simulink model "BANSHEE"  (Simulink 8.1)
settings: Solver=ode1  StartTime=0.0  StopTime=inf  FixedStep=Ts  MaxStep=1e-3  RelTol=1e-3
PostLoadFcn:
  | BANSHEE_init;
InitFcn:
  | BANSHEE_init;
undefined symbols (not defined in the file): Acid, Banshee_HWCtrl_IOs, Banshee_SEL751_Woodward_lib, DMS_slave_lib, DMSCommands, F1, F2, F3, fdesignblkfcn, Feeder1_lib, Feeder2_lib, Feeder3_lib, gcbh, generic_ethernet_cb, Lead, Left, relay_housing_lib, SM_UtilityService, SS_F1_RELAY_HOUSING, SS_F2_RELAY_HOUSING, SS_F3_RELAY_HOUSING, SS_Feeder1, SS_Feeder2, SS_Feeder3, SUBSTATION, TestSeq_slave_lib, TestSequenceCommands, Ts, type, utility_service_lib, V
libraries: powerlib x106, cables_lib x61, breaker_lib x53, rtio_generic_modbus x50, relay_modbus_lib x45, rtio_opalrt_op5142ex1 x37, transformer_lib x29, rteventslib x28, simulink x24, Load_lib x24, rtlab x20, ssn_lib x19
(part 8 of 9)

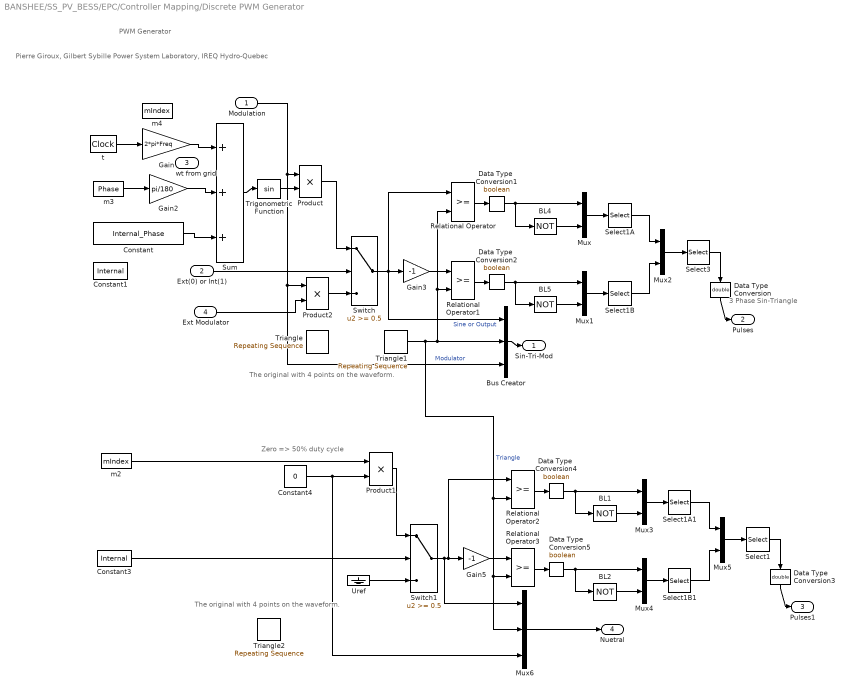
== system BANSHEE/SS_PV_BESS/EPC/Controller Mapping/Discrete PWM Generator ==
  note: Pierre Giroux, Gilbert Sybille
      | Power System Laboratory, IREQ
      | Hydro-Quebec
  note: PWM Generator
  note: 3 Phase
      | Sin-Triangle
  note: Zero => 50% duty cycle
  note: The original with 4
      | points on the waveform.
  note: The original with 4
      | points on the waveform.
  Modulation : Inport
  Ext(0) or Int(1) : Inport  Port=2
  wt from grid : Inport  Port=3
  Ext Modulator : Inport  Port=4
  BL{1..2,4..5} (4 alike) : Logic  Operator=NOT  Inputs=1  SampleTime=Ts
  Bus Creator : BusCreator  Inputs=3
  Constant : Constant  Value=Internal_Phase  SampleTime=Ts
  Constant1 : Constant  Value=Internal  SampleTime=Ts
  Constant3 : Constant  Value=Internal  SampleTime=Ts
  Constant4 : Constant  Value=0
  Data Type  Conversion : DataTypeConversion  OutDataTypeStr=double  SampleTime=Ts  SaturateOnIntegerOverflow=on  RndMeth=Zero
  Data Type  Conversion{1..2,4..5} (4 alike) : DataTypeConversion  OutDataTypeStr=boolean  SampleTime=Ts  SaturateOnIntegerOverflow=on  RndMeth=Zero
  Data Type  Conversion3 : DataTypeConversion  OutDataTypeStr=double  SampleTime=Ts  SaturateOnIntegerOverflow=on  RndMeth=Zero
  Gain : Gain  Gain=2*pi*Freq  SaturateOnIntegerOverflow=on  OutDataTypeStr=Inherit: Same as input  ParamDataTypeStr=Inherit: Same as input
  Gain2 : Gain  Gain=pi/180  SaturateOnIntegerOverflow=on  OutDataTypeStr=Inherit: Same as input  ParamDataTypeStr=Inherit: Same as input
  Gain3 : Gain  Gain=-1  SampleTime=Ts  SaturateOnIntegerOverflow=on  OutDataTypeStr=Inherit: Same as input  ParamDataTypeStr=Inherit: Same as input
  Gain5 : Gain  Gain=-1  SampleTime=Ts  SaturateOnIntegerOverflow=on  OutDataTypeStr=Inherit: Same as input  ParamDataTypeStr=Inherit: Same as input
  Mux{,1..5} (6 alike) : Mux  Inputs=2
  Mux6 : Mux  Inputs=3
  Product : Product  SampleTime=Ts  SaturateOnIntegerOverflow=on  InputSameDT=on  OutDataTypeStr=Inherit: Same as first input
  Product1 : Product  SampleTime=Ts  SaturateOnIntegerOverflow=on  InputSameDT=on  OutDataTypeStr=Inherit: Same as first input
  Product2 : Product  SampleTime=Ts  SaturateOnIntegerOverflow=on  InputSameDT=on  OutDataTypeStr=Inherit: Same as first input
  Relational Operator{,1..3} (4 alike) : RelationalOperator  SampleTime=Ts  InputSameDT=on
  Select1 : Selector  InputPortWidth=Select3_PortWidth  IndexOptions=Index vector (dialog)  Indices=Select3_Elements  OutputSizes=1
  Select1A : Selector  InputPortWidth=Select1_PortWidth  IndexOptions=Index vector (dialog)  Indices=Select1_Elements  OutputSizes=1
  Select1A1 : Selector  InputPortWidth=Select1_PortWidth  IndexOptions=Index vector (dialog)  Indices=Select1_Elements  OutputSizes=1
  Select1B : Selector  InputPortWidth=Select1_PortWidth  IndexOptions=Index vector (dialog)  Indices=Select1_Elements  OutputSizes=1
  Select1B1 : Selector  InputPortWidth=Select1_PortWidth  IndexOptions=Index vector (dialog)  Indices=Select1_Elements  OutputSizes=1
  Select3 : Selector  InputPortWidth=Select3_PortWidth  IndexOptions=Index vector (dialog)  Indices=Select3_Elements  OutputSizes=1
  Sum : Sum  Inputs=+++  SampleTime=Ts  SaturateOnIntegerOverflow=on  InputSameDT=on  OutDataTypeStr=Inherit: Same as first input
  Switch : Switch  Threshold=0.5  SampleTime=Ts  SaturateOnIntegerOverflow=on  InputSameDT=on
  Switch1 : Switch  Threshold=0.5  SampleTime=Ts  SaturateOnIntegerOverflow=on  InputSameDT=on
  Triangle : simulink/Sources/Repeating Sequence  rep_seq_t=[0 1/Fc/4 3/Fc/4 1/Fc]  rep_seq_y=[0 -1 1 0]
  Triangle1 : simulink/Sources/Repeating Sequence  rep_seq_t=[0 1/Fc/2 1/Fc]  rep_seq_y=[-1 1 -1]
  Triangle2 : simulink/Sources/Repeating Sequence  rep_seq_t=[0 1/Fc/4 3/Fc/4 1/Fc]  rep_seq_y=[0 -1 1 0]
  Trigonometric Function : Trigonometry  SampleTime=Ts
  Uref : Ground
  m2 : Constant  Value=mIndex  SampleTime=Ts
  m3 : Constant  Value=Phase  SampleTime=Ts
  m4 : Constant  Value=mIndex  SampleTime=Ts
  t : DigitalClock  SampleTime=Ts
  Sin-Tri-Mod : Outport  SampleTime=Ts
  Pulses : Outport  Port=2  SampleTime=Ts
  Pulses1 : Outport  Port=3  SampleTime=Ts
  Nuetral : Outport  Port=4  SampleTime=Ts
  wires:
  Switch/1 -> Relational Operator/1, Gain3/1, Bus Creator/1  "Sine or Output"
  Mux2/1 -> Select3/1
  Select1B/1 -> Mux2/2
  Select1A/1 -> Mux2/1
  Mux1/1 -> Select1B/1
  Mux/1 -> Select1A/1
  BL5/1 -> Mux1/2
  BL4/1 -> Mux/2
  Gain3/1 -> Relational Operator1/1
  Product/1 -> Switch/1
  Trigonometric Function/1 -> Product/2
  Sum/1 -> Trigonometric Function/1
  m3/1 -> Gain2/1
  t/1 -> Gain/1
  Select3/1 -> Data Type  Conversion/1
  Data Type  Conversion/1 -> Pulses/1
  Relational Operator/1 -> Data Type  Conversion1/1
  Data Type  Conversion1/1 -> BL4/1, Mux/1
  Relational Operator1/1 -> Data Type  Conversion2/1
  Data Type  Conversion2/1 -> BL5/1, Mux1/1
  Bus Creator/1 -> Sin-Tri-Mod/1
  Triangle1/1 -> Bus Creator/2, Relational Operator1/2, Relational Operator/2, Relational Operator3/2, Mux6/2, Relational Operator2/2  "Triangle"
  Switch1/1 -> Relational Operator2/1, Gain5/1, Mux6/1
  Mux5/1 -> Select1/1
  Select1B1/1 -> Mux5/2
  Select1A1/1 -> Mux5/1
  Mux4/1 -> Select1B1/1
  Mux3/1 -> Select1A1/1
  BL2/1 -> Mux4/2
  BL1/1 -> Mux3/2
  Gain5/1 -> Relational Operator3/1
  Product1/1 -> Switch1/1
  m2/1 -> Product1/1
  Select1/1 -> Data Type  Conversion3/1
  Data Type  Conversion3/1 -> Pulses1/1
  Relational Operator2/1 -> Data Type  Conversion4/1
  Data Type  Conversion4/1 -> BL1/1, Mux3/1
  Relational Operator3/1 -> Data Type  Conversion5/1
  Data Type  Conversion5/1 -> BL2/1, Mux4/1
  Constant4/1 -> Product1/2, Mux6/3
  Mux6/1 -> Nuetral/1
  Product2/1 -> Switch/3
  Constant3/1 -> Switch1/2
  Uref/1 -> Switch1/3
  Ext(0) or Int(1)/1 -> Switch/2
  Modulation/1 -> Bus Creator/3, Product2/1, Product/1  "Modulator"
  Ext Modulator/1 -> Product2/2
  Constant/1 -> Sum/3
  Gain2/1 -> Sum/2
  Gain/1 -> Sum/1

== system BANSHEE/SS_PV_BESS/EPC/Controller Mapping/EPC Inverter Controller Outputs ==
  note: These PWM IN Signals will be used.
      | PWM 1 and 2 are Bot and Top
      | PWM 3 and 4 are Bot and Top
      | PWM 5 and 6 are Bot and Top
  note: When using TSD set the DOUT type config to 0
      | When using PWM set the DOUT type config to 1
  note: It was at 1 for PWM, but it seems that
      | it is better to use the event detector conversion
      | block with TSD instead.
  note: % Copyright (c) 2016 Massachusetts Institute of Technology
      | % Permission is hereby granted, free of charge, to any person obtaining a copy of this
      | % software and associated documentation files (the "Software"), to deal in the Software
      | % without restriction, including without limitation the rights to use, copy, modify,
      | % merge, publish, distribute, sublicense, and/or sell copies of the Software, and to
      | % permit persons to whom the Software is furnished to do so, subject to the following
      | % conditions:
      | %
      | %
      | % The above copyright notice and this permission notice shall be included in
      | % all copies or substantial portions of the Software.
      | %
      | % THE SOFTWARE IS PROVIDED "AS IS", WITHOUT WARRANTY OF ANY KIND, EXPRESS OR IMPLIED,
      | % INCLUDING BUT NOT LIMITED TO THE WARRANTIES OF MERCHANTABILITY, FITNESS FOR A
      | % PARTICULAR PURPOSE AND NONINFRINGEMENT. IN NO EVENT SHALL THE AUTHORS OR COPYRIGHT
      | % HOLDERS BE LIABLE FOR ANY CLAIM, DAMAGES OR OTHER LIABILITY, WHETHER IN AN ACTION
      | % OF CONTRACT, TORT OR OTHERWISE, ARISING FROM, OUT OF OR IN CONNECTION WITH THE
      | % SOFTWARE OR THE USE OR OTHER DEALINGS IN THE SOFTWARE.
      | %
      | %
      | %%
  Console Input : Inport
  Bus Creator1 : BusCreator  Inputs=3
  Bus Creator2 : BusCreator  Inputs=2
  Bus Selector1 : BusSelector  OutputSignals=00-03,04-07  OutputAsBus=on
  Bus Selector2 : BusSelector  OutputSignals=08-11,12-15  OutputAsBus=on
  Bus Selector6 : BusSelector  OutputSignals=16 DOUT GR3,16 TSDOUT GR3,16 PWMOUT GR3
  DIO - Gr4 : Subsystem
  DOUT type config : Subsystem
  GR1 B AIN (CH00-15) : Subsystem
  OpCtrl OP5142EX2 : rtio_opalrt_op5142ex1/OpCtrl OP5142EX1  CtrlName='OP5142EX2 Ctrl'  boardid=2  BitstreamFilename=OP5142_1-EX-0000-2_3_4_54-16AIO_48AO_16DIO_16selDIO_CD-FF-01.bin  numconfig=-1  mode=Slave  externalClock=off  decimRtsi=0  calibIO=off  SampleTime=0  loadinport=-1
  PWM IO - Gr4 : Subsystem
  TSDIO - Gr4 : Subsystem
  Error : Outport
  IDs : Outport  Port=2
  PWM : Outport  Port=3
  Digital Inputs : Outport  Port=4
  PWM_RTE : Outport  Port=5
  BESS_TSD_RTE : Outport  Port=6
  PV_TSD_RTE : Outport  Port=7
  wires:
  TSDIO - Gr4/3(PV_TSDin_RTE) -> PV_TSD_RTE/1
  OpCtrl OP5142EX2/1 -> Error/1
  OpCtrl OP5142EX2/2 -> IDs/1
  PWM IO - Gr4/1(PWMIn) -> Bus Creator1/3, PWM/1  "PWMIN"
  TSDIO - Gr4/1(TSDin) -> Bus Creator1/2  "TSDIN"
  DIO - Gr4/1(DIn) -> Bus Creator1/1  "DIN"
  Bus Creator1/1 -> Digital Inputs/1
  Console Input/1 -> Bus Selector6/1
  Bus Selector6/2 -> TSDIO - Gr4/1(TSDout)  "<16 TSDOUT GR3>"
  Bus Selector6/3 -> PWM IO - Gr4/1(PWMOut)  "<16 PWMOUT GR3>"
  Bus Selector6/1 -> Bus Selector1/1, Bus Selector2/1  "<16 DOUT GR3>"
  Bus Selector1/1 -> Bus Creator2/1  "DI_CH00-07"
  Bus Selector2/1 -> Bus Creator2/2  "DI_CH08-15"
  Bus Creator2/1 -> DIO - Gr4/1(Dout)
  PWM IO - Gr4/2(PWMIn_RTE) -> PWM_RTE/1
  TSDIO - Gr4/2(BESS_TSDin_RTE) -> BESS_TSD_RTE/1

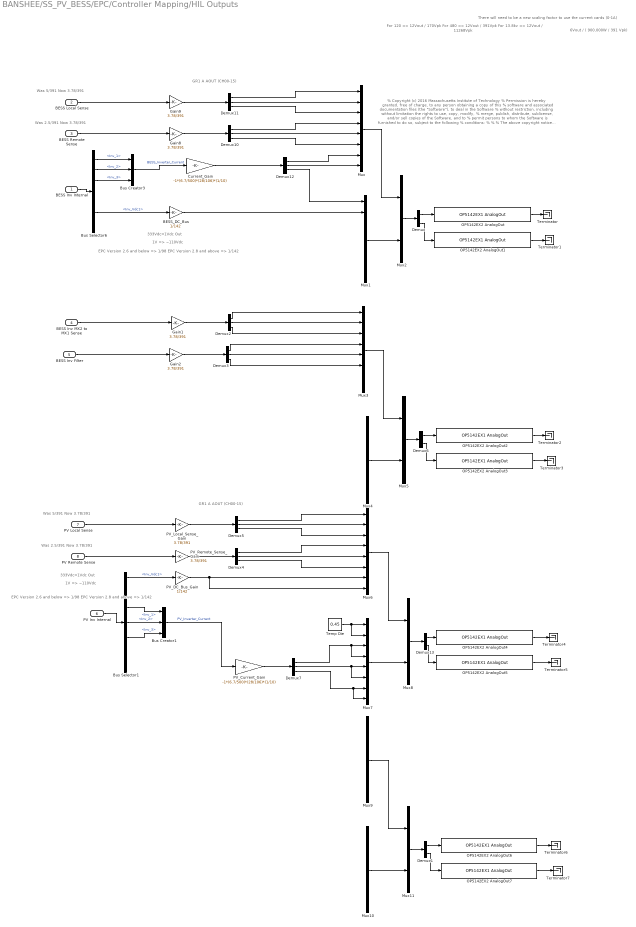
== system BANSHEE/SS_PV_BESS/EPC/Controller Mapping/HIL Outputs ==
  note: GR1 A AOUT (CH00-15)
  note: 333Vdc=1Vdc Out
  note: 1V => ~110Vdc
  note: Was 5/391
      | Now 3.78/391
  note: Was 2.5/391
      | Now 3.78/391
  note: EPC Version 2.6 and below => 1/98
      | EPC Version 2.8 and above => 1/142
  note: 6Vout / ( 900,000W / 391 Vpk)
  note: For 120 => 12Vout / 170Vpk
      | For 480 => 12Vout / 391Vpk
      | For 13.8kv => 12Vout / 11268Vpk
  note: GR1 A AOUT (CH00-15)
  note: There will need to be a
      | new scaling factor to use
      | the current cards (0-1A)
  note: 333Vdc=1Vdc Out
  note: 1V => ~110Vdc
  note: Was 5/391
      | Now 3.78/391
  note: Was 2.5/391
      | Now 3.78/391
  note: EPC Version 2.6 and below => 1/98
      | EPC Version 2.8 and above => 1/142
  note: % Copyright (c) 2016 Massachusetts Institute of Technology
      | % Permission is hereby granted, free of charge, to any person obtaining a copy of this
      | % software and associated documentation files (the "Software"), to deal in the Software
      | % without restriction, including without limitation the rights to use, copy, modify,
      | % merge, publish, distribute, sublicense, and/or sell copies of the Software, and to
      | % permit persons to whom the Software is furnished to do so, subject to the following
      | % conditions:
      | %
      | %
      | % The above copyright notice and this permission notice shall be included in
      | % all copies or substantial portions of the Software.
      | %
      | % THE SOFTWARE IS PROVIDED "AS IS", WITHOUT WARRANTY OF ANY KIND, EXPRESS OR IMPLIED,
      | % INCLUDING BUT NOT LIMITED TO THE WARRANTIES OF MERCHANTABILITY, FITNESS FOR A
      | % PARTICULAR PURPOSE AND NONINFRINGEMENT. IN NO EVENT SHALL THE AUTHORS OR COPYRIGHT
      | % HOLDERS BE LIABLE FOR ANY CLAIM, DAMAGES OR OTHER LIABILITY, WHETHER IN AN ACTION
      | % OF CONTRACT, TORT OR OTHERWISE, ARISING FROM, OUT OF OR IN CONNECTION WITH THE
      | % SOFTWARE OR THE USE OR OTHER DEALINGS IN THE SOFTWARE.
      | %
      | %
      | %%
  BESS Inv Internal : Inport
  BESS Local Sense : Inport  Port=2
  BESS Remote Sense : Inport  Port=3
  BESS Inv MX2 to MX1 Sense : Inport  Port=4
  BESS Inv Filter : Inport  Port=5
  PV Inv Internal : Inport  Port=6
  PV Local Sense : Inport  Port=7
  PV Remote Sense : Inport  Port=8
  BESS_DC_Bus : Gain  Gain=1/142
  Bus Creator1 : BusCreator  Inputs=3
  Bus Creator3 : BusCreator  Inputs=3
  Bus Selector1 : BusSelector  OutputSignals=Inv_Vdc1,Inv_Vdc2,Inv_1,Inv_2,Inv_3,Inv_Idc1,Inv_Idc2
  Bus Selector6 : BusSelector  OutputSignals=Inv_1,Inv_2,Inv_3,Inv_Idc1,Inv_Idc2,Inv_Vdc1,Inv_Vdc2
  Current_Gain : Gain  Gain=-1*(6.7/500)*(28/106)*(1/10)
  Demux{,1,6,13} (4 alike) : Demux  Outputs=2
  Demux{2..5,7,10..12} (8 alike) : Demux  Outputs=3
  Gain{1..2,8..9} (4 alike) : Gain  Gain=3.78/391
  Mux{,1,3..4,6..7,9..10} (8 alike) : Mux  Inputs=8
  Mux{2,5,8,11} (4 alike) : Mux  Inputs=2
  OP5142EX2 AnalogOut : rtio_opalrt_op5142ex1/OP5142EX1 AnalogOut  CtrlName='OP5142EX2 Ctrl'  portNb=1  FcnNos=Slot 1 Module A Subsection 1  size=16  maxcount=8  count=8  numchan=8  israngeinput=off  voltagerange=[-16 ... 16]  slot=0  side=0  mismatch=0  slotside=Slot_1_Module_A
      settings: AttributesFormatString=%<CtrlName>
  OP5142EX2 AnalogOut1 : rtio_opalrt_op5142ex1/OP5142EX1 AnalogOut  CtrlName='OP5142EX2 Ctrl'  portNb=2  FcnNos=Slot 1 Module A Subsection 2  size=16  maxcount=8  count=8  numchan=8  israngeinput=off  voltagerange=[-16 ... 16]  slot=0  side=0  mismatch=0  slotside=Slot_1_Module_A
      settings: AttributesFormatString=%<CtrlName>
  OP5142EX2 AnalogOut2 : rtio_opalrt_op5142ex1/OP5142EX1 AnalogOut  CtrlName='OP5142EX2 Ctrl'  portNb=3  FcnNos=Slot 2 Module A Subsection 1  size=16  maxcount=8  count=8  numchan=8  israngeinput=off  voltagerange=[-16 ... 16]  slot=1  side=0  mismatch=0  slotside=Slot_2_Module_A
      settings: AttributesFormatString=%<CtrlName>
  OP5142EX2 AnalogOut3 : rtio_opalrt_op5142ex1/OP5142EX1 AnalogOut  CtrlName='OP5142EX2 Ctrl'  portNb=4  FcnNos=Slot 2 Module A Subsection 2  size=16  maxcount=8  count=8  numchan=8  israngeinput=off  voltagerange=[-16 ... 16]  slot=1  side=0  mismatch=0  slotside=Slot_2_Module_A
      settings: AttributesFormatString=%<CtrlName>
  OP5142EX2 AnalogOut4 : rtio_opalrt_op5142ex1/OP5142EX1 AnalogOut  CtrlName='OP5142EX2 Ctrl'  portNb=5  FcnNos=Slot 2 Module B Subsection 1  size=16  maxcount=8  count=8  numchan=8  israngeinput=off  voltagerange=[-16 ... 16]  slot=1  side=1  mismatch=0  slotside=Slot_2_Module_B
      settings: AttributesFormatString=%<CtrlName>
  OP5142EX2 AnalogOut5 : rtio_opalrt_op5142ex1/OP5142EX1 AnalogOut  CtrlName='OP5142EX2 Ctrl'  portNb=6  FcnNos=Slot 2 Module B Subsection 2  size=16  maxcount=8  count=8  numchan=8  israngeinput=off  voltagerange=[-16 ... 16]  slot=1  side=1  mismatch=0  slotside=Slot_2_Module_B
      settings: AttributesFormatString=%<CtrlName>
  OP5142EX2 AnalogOut6 : rtio_opalrt_op5142ex1/OP5142EX1 AnalogOut  CtrlName='OP5142EX2 Ctrl'  portNb=7  FcnNos=Slot 3 Module A Subsection 1  size=16  maxcount=8  count=8  numchan=8  israngeinput=off  voltagerange=[-16 ... 16]  slot=2  side=0  mismatch=0  slotside=Slot_3_Module_A
      settings: AttributesFormatString=%<CtrlName>
  OP5142EX2 AnalogOut7 : rtio_opalrt_op5142ex1/OP5142EX1 AnalogOut  CtrlName='OP5142EX2 Ctrl'  portNb=8  FcnNos=Slot 3 Module A Subsection 2  size=16  maxcount=8  count=8  numchan=8  israngeinput=off  voltagerange=[-16 ... 16]  slot=2  side=0  mismatch=0  slotside=Slot_3_Module_A
      settings: AttributesFormatString=%<CtrlName>
  PV_Current_Gain : Gain  Gain=-1*(6.7/500)*(28/106)*(1/10)
  PV_DC_Bus_Gain : Gain  Gain=1/142
  PV_Local_Sense_Gain : Gain  Gain=3.78/391
  PV_Remote_Sense_Gain : Gain  Gain=3.78/391
  Temp Die : Constant  Value=0.45
  Terminator{,1..7} (8 alike) : Terminator
  wires:
  Temp Die/1 -> Mux7/1, Mux7/2
  Demux7/3 -> Mux7/7, Mux7/8
  Demux7/2 -> Mux7/5, Mux7/6
  Demux7/1 -> Mux7/3, Mux7/4
  Demux4/3 -> Mux6/6
  Demux4/1 -> Mux6/4
  Demux4/2 -> Mux6/5
  Demux5/3 -> Mux6/3
  Demux5/1 -> Mux6/1
  Demux5/2 -> Mux6/2
  PV_Current_Gain/1 -> Demux7/1
  PV_Remote_Sense_Gain/1 -> Demux4/1
  PV_Local_Sense_Gain/1 -> Demux5/1
  PV_DC_Bus_Gain/1 -> Mux6/8, Mux6/7
  PV Inv Internal/1 -> Bus Selector1/1
  PV Local Sense/1 -> PV_Local_Sense_Gain/1
  PV Remote Sense/1 -> PV_Remote_Sense_Gain/1
  Bus Creator1/1 -> PV_Current_Gain/1  "PV_Inverter_Current"
  Bus Selector1/3 -> Bus Creator1/1  "<Inv_1>"
  Bus Selector1/4 -> Bus Creator1/2  "<Inv_2>"
  Bus Selector1/5 -> Bus Creator1/3  "<Inv_3>"
  Bus Selector1/1 -> PV_DC_Bus_Gain/1  "<Inv_Vdc1>"
  Demux10/3 -> Mux/6
  Demux10/1 -> Mux/4
  Demux10/2 -> Mux/5
  Demux11/3 -> Mux/3
  Demux11/1 -> Mux/1
  Demux11/2 -> Mux/2
  Current_Gain/1 -> Demux12/1
  Mux2/1 -> Demux/1
  Mux1/1 -> Mux2/2
  Mux/1 -> Mux2/1
  Demux/2 -> OP5142EX2 AnalogOut1/1
  Demux/1 -> OP5142EX2 AnalogOut/1
  OP5142EX2 AnalogOut1/1 -> Terminator1/1
  OP5142EX2 AnalogOut/1 -> Terminator/1
  Mux5/1 -> Demux6/1
  Mux4/1 -> Mux5/2
  Mux3/1 -> Mux5/1
  Demux6/2 -> OP5142EX2 AnalogOut3/1
  Demux6/1 -> OP5142EX2 AnalogOut2/1
  OP5142EX2 AnalogOut3/1 -> Terminator3/1
  OP5142EX2 AnalogOut2/1 -> Terminator2/1
  Mux8/1 -> Demux13/1
  Mux7/1 -> Mux8/2
  Mux6/1 -> Mux8/1
  Gain8/1 -> Demux10/1
  Gain9/1 -> Demux11/1
  BESS_DC_Bus/1 -> Mux1/2
  BESS Inv Internal/1 -> Bus Selector6/1
  BESS Local Sense/1 -> Gain9/1
  BESS Remote Sense/1 -> Gain8/1
  Bus Creator3/1 -> Current_Gain/1  "BESS_Inverter_Current"
  Demux12/1 -> Mux/7
  Demux12/2 -> Mux/8
  Demux12/3 -> Mux1/1
  Bus Selector6/1 -> Bus Creator3/1  "<Inv_1>"
  Bus Selector6/2 -> Bus Creator3/2  "<Inv_2>"
  Bus Selector6/3 -> Bus Creator3/3  "<Inv_3>"
  Bus Selector6/6 -> BESS_DC_Bus/1  "<Inv_Vdc1>"
  Mux11/1 -> Demux1/1
  Mux10/1 -> Mux11/2
  Mux9/1 -> Mux11/1
  Demux13/1 -> OP5142EX2 AnalogOut4/1
  Demux13/2 -> OP5142EX2 AnalogOut5/1
  OP5142EX2 AnalogOut4/1 -> Terminator4/1
  OP5142EX2 AnalogOut5/1 -> Terminator5/1
  Demux1/1 -> OP5142EX2 AnalogOut6/1
  Demux1/2 -> OP5142EX2 AnalogOut7/1
  OP5142EX2 AnalogOut6/1 -> Terminator6/1
  OP5142EX2 AnalogOut7/1 -> Terminator7/1
  Gain1/1 -> Demux2/1
  BESS Inv MX2 to MX1 Sense/1 -> Gain1/1
  Demux2/1 -> Mux3/1
  Demux2/2 -> Mux3/2
  Demux2/3 -> Mux3/3
  Gain2/1 -> Demux3/1
  BESS Inv Filter/1 -> Gain2/1
  Demux3/1 -> Mux3/4
  Demux3/2 -> Mux3/5
  Demux3/3 -> Mux3/6

== system BANSHEE/SS_PV_BESS/EPC/Controller Mapping/Mux to Pulses1 ==
  Mux_6_Pulses : Inport
  Bus Creator24 : BusCreator  Inputs=6
  Bus Selector5 : BusSelector  OutputSignals=Pulse 1,Pulse 2,Pulse 3,Pulse 4,Pulse 5,Pulse 6
  Demux5 : Demux  Outputs=6
  Pulse1 : Outport
  Pulse2 : Outport  Port=2
  Pulse3 : Outport  Port=3
  Pulse4 : Outport  Port=4
  Pulse5 : Outport  Port=5
  Pulse6 : Outport  Port=6
  Bus : Outport  Port=7
  wires:
  Demux5/1 -> Bus Creator24/1  "Pulse 1"
  Demux5/2 -> Bus Creator24/2  "Pulse 2"
  Demux5/3 -> Bus Creator24/3  "Pulse 3"
  Demux5/4 -> Bus Creator24/4  "Pulse 4"
  Demux5/5 -> Bus Creator24/5  "Pulse 5"
  Demux5/6 -> Bus Creator24/6  "Pulse 6"
  Bus Creator24/1 -> Bus Selector5/1, Bus/1
  Mux_6_Pulses/1 -> Demux5/1
  Bus Selector5/1 -> Pulse1/1  "<Pulse 1>"
  Bus Selector5/2 -> Pulse2/1  "<Pulse 2>"
  Bus Selector5/3 -> Pulse3/1  "<Pulse 3>"
  Bus Selector5/4 -> Pulse4/1  "<Pulse 4>"
  Bus Selector5/5 -> Pulse5/1  "<Pulse 5>"
  Bus Selector5/6 -> Pulse6/1  "<Pulse 6>"

== system BANSHEE/SS_PV_BESS/EPC/Controller Mapping/Mux to Pulses2 ==
  Mux_6_Pulses : Inport
  Bus Creator24 : BusCreator  Inputs=6
  Bus Selector5 : BusSelector  OutputSignals=Pulse 1,Pulse 2,Pulse 3,Pulse 4,Pulse 5,Pulse 6
  Demux5 : Demux  Outputs=6
  Pulse1 : Outport
  Pulse2 : Outport  Port=2
  Pulse3 : Outport  Port=3
  Pulse4 : Outport  Port=4
  Pulse5 : Outport  Port=5
  Pulse6 : Outport  Port=6
  Bus : Outport  Port=7
  wires:
  Demux5/1 -> Bus Creator24/1  "Pulse 1"
  Demux5/2 -> Bus Creator24/2  "Pulse 2"
  Demux5/3 -> Bus Creator24/3  "Pulse 3"
  Demux5/4 -> Bus Creator24/4  "Pulse 4"
  Demux5/5 -> Bus Creator24/5  "Pulse 5"
  Demux5/6 -> Bus Creator24/6  "Pulse 6"
  Bus Creator24/1 -> Bus Selector5/1, Bus/1
  Mux_6_Pulses/1 -> Demux5/1
  Bus Selector5/1 -> Pulse1/1  "<Pulse 1>"
  Bus Selector5/2 -> Pulse2/1  "<Pulse 2>"
  Bus Selector5/3 -> Pulse3/1  "<Pulse 3>"
  Bus Selector5/4 -> Pulse4/1  "<Pulse 4>"
  Bus Selector5/5 -> Pulse5/1  "<Pulse 5>"
  Bus Selector5/6 -> Pulse6/1  "<Pulse 6>"

== system BANSHEE/SS_PV_BESS/EPC/Controller Mapping/Mux to Pulses3 ==
  Mux_6_Pulses : Inport
  Bus Creator24 : BusCreator  Inputs=6
  Bus Selector5 : BusSelector  OutputSignals=Pulse 1,Pulse 2,Pulse 3,Pulse 4,Pulse 5,Pulse 6
  Demux5 : Demux  Outputs=6
  Pulse1 : Outport
  Pulse2 : Outport  Port=2
  Pulse3 : Outport  Port=3
  Pulse4 : Outport  Port=4
  Pulse5 : Outport  Port=5
  Pulse6 : Outport  Port=6
  Bus : Outport  Port=7
  wires:
  Demux5/1 -> Bus Creator24/1  "Pulse 1"
  Demux5/2 -> Bus Creator24/2  "Pulse 2"
  Demux5/3 -> Bus Creator24/3  "Pulse 3"
  Demux5/4 -> Bus Creator24/4  "Pulse 4"
  Demux5/5 -> Bus Creator24/5  "Pulse 5"
  Demux5/6 -> Bus Creator24/6  "Pulse 6"
  Bus Creator24/1 -> Bus Selector5/1, Bus/1
  Mux_6_Pulses/1 -> Demux5/1
  Bus Selector5/1 -> Pulse1/1  "<Pulse 1>"
  Bus Selector5/2 -> Pulse2/1  "<Pulse 2>"
  Bus Selector5/3 -> Pulse3/1  "<Pulse 3>"
  Bus Selector5/4 -> Pulse4/1  "<Pulse 4>"
  Bus Selector5/5 -> Pulse5/1  "<Pulse 5>"
  Bus Selector5/6 -> Pulse6/1  "<Pulse 6>"

== system BANSHEE/SS_PV_BESS/EPC/Controller Mapping/Mux to Pulses4 ==
  Mux_6_Pulses : Inport
  Bus Creator24 : BusCreator  Inputs=6
  Bus Selector5 : BusSelector  OutputSignals=Pulse 1,Pulse 2,Pulse 3,Pulse 4,Pulse 5,Pulse 6
  Demux5 : Demux  Outputs=6
  Pulse1 : Outport
  Pulse2 : Outport  Port=2
  Pulse3 : Outport  Port=3
  Pulse4 : Outport  Port=4
  Pulse5 : Outport  Port=5
  Pulse6 : Outport  Port=6
  Bus : Outport  Port=7
  wires:
  Demux5/1 -> Bus Creator24/1  "Pulse 1"
  Demux5/2 -> Bus Creator24/2  "Pulse 2"
  Demux5/3 -> Bus Creator24/3  "Pulse 3"
  Demux5/4 -> Bus Creator24/4  "Pulse 4"
  Demux5/5 -> Bus Creator24/5  "Pulse 5"
  Demux5/6 -> Bus Creator24/6  "Pulse 6"
  Bus Creator24/1 -> Bus Selector5/1, Bus/1
  Mux_6_Pulses/1 -> Demux5/1
  Bus Selector5/1 -> Pulse1/1  "<Pulse 1>"
  Bus Selector5/2 -> Pulse2/1  "<Pulse 2>"
  Bus Selector5/3 -> Pulse3/1  "<Pulse 3>"
  Bus Selector5/4 -> Pulse4/1  "<Pulse 4>"
  Bus Selector5/5 -> Pulse5/1  "<Pulse 5>"
  Bus Selector5/6 -> Pulse6/1  "<Pulse 6>"

== system BANSHEE/SS_PV_BESS/EPC/Controller Mapping/Mux to Pulses5 ==
  Mux_6_Pulses : Inport
  Bus Creator24 : BusCreator  Inputs=6
  Bus Selector5 : BusSelector  OutputSignals=Pulse 1,Pulse 2,Pulse 3,Pulse 4,Pulse 5,Pulse 6
  Demux5 : Demux  Outputs=6
  Pulse1 : Outport
  Pulse2 : Outport  Port=2
  Pulse3 : Outport  Port=3
  Pulse4 : Outport  Port=4
  Pulse5 : Outport  Port=5
  Pulse6 : Outport  Port=6
  Bus : Outport  Port=7
  wires:
  Demux5/1 -> Bus Creator24/1  "Pulse 1"
  Demux5/2 -> Bus Creator24/2  "Pulse 2"
  Demux5/3 -> Bus Creator24/3  "Pulse 3"
  Demux5/4 -> Bus Creator24/4  "Pulse 4"
  Demux5/5 -> Bus Creator24/5  "Pulse 5"
  Demux5/6 -> Bus Creator24/6  "Pulse 6"
  Bus Creator24/1 -> Bus Selector5/1, Bus/1
  Mux_6_Pulses/1 -> Demux5/1
  Bus Selector5/1 -> Pulse1/1  "<Pulse 1>"
  Bus Selector5/2 -> Pulse2/1  "<Pulse 2>"
  Bus Selector5/3 -> Pulse3/1  "<Pulse 3>"
  Bus Selector5/4 -> Pulse4/1  "<Pulse 4>"
  Bus Selector5/5 -> Pulse5/1  "<Pulse 5>"
  Bus Selector5/6 -> Pulse6/1  "<Pulse 6>"

== system BANSHEE/SS_PV_BESS/EPC/Controller Mapping/Open Top ==
  note: This is for the Gate Drive RTE block. The block does
      | not allow for all the switches to be open at the same time.
  Bus Creator18 : BusCreator  Inputs=6
  GD1_1 : Constant  Value=0
  GD1_2 : Constant
  RTE Conversion2 : rteventslib/Signal Attributes/RTE Conversion  inputdatatype=Double  outputdatatype=RTE Boolean  compensation=Disabled  nbMaxEvents=4  sampleTime=Ts
  Pulses6 : Outport
  wires:
  GD1_1/1 -> Bus Creator18/2, Bus Creator18/6, Bus Creator18/4
  Bus Creator18/1 -> RTE Conversion2/1
  RTE Conversion2/1 -> Pulses6/1
  GD1_2/1 -> Bus Creator18/1, Bus Creator18/3, Bus Creator18/5

== system BANSHEE/SS_PV_BESS/EPC/Controller Mapping/PV Signal Mapping ==
  In1 : Inport
  Bus Creator1 : BusCreator  Inputs=6
  Demux1 : Demux  Outputs=6
  TSD_RTE_v2 : Outport
  wires:
  In1/1 -> Demux1/1
  Bus Creator1/1 -> TSD_RTE_v2/1
  Demux1/6 -> Bus Creator1/6  "Phase 3 Bottom"
  Demux1/5 -> Bus Creator1/5  "Phase 3 Top"
  Demux1/4 -> Bus Creator1/4  "Phase 2 Bottom"
  Demux1/3 -> Bus Creator1/3  "Phase 2 Top"
  Demux1/2 -> Bus Creator1/2  "Phase 1 Bottom"
  Demux1/1 -> Bus Creator1/1  "Phase 1 Top"

== system BANSHEE/SS_PV_BESS/EPC/Controller Mapping/PWM to RTE PWM ==
  note: Can one block if mapped
      | or muxed correctly do all
      | of these signals?
      |
      | Check that the correct signal
      | goes to the correct gate.
  PWM_in : Inport
  Bus Creator : BusCreator  Inputs=6
  Bus Selector3 : BusSelector  OutputSignals=PWMIN.PWMI_CH16-23.Freq,PWMIN.PWMI_CH16-23.Duty
  Demux : Demux  Outputs=8
  Demux2 : Demux  Outputs=8
  RTE PWM Bot 1 : rteventslib/Sources/RTE PWM  ShiftedTransition=Enabled  MaxEvents=4  SampleTime=Ts
  RTE PWM Bot 2 : rteventslib/Sources/RTE PWM  ShiftedTransition=Enabled  MaxEvents=4  SampleTime=Ts
  RTE PWM Bot 3 : rteventslib/Sources/RTE PWM  ShiftedTransition=Enabled  MaxEvents=4  SampleTime=Ts
  RTE PWM Top 1 : rteventslib/Sources/RTE PWM  ShiftedTransition=Enabled  MaxEvents=4  SampleTime=Ts
  RTE PWM Top 2 : rteventslib/Sources/RTE PWM  ShiftedTransition=Enabled  MaxEvents=4  SampleTime=Ts
  RTE PWM Top 3 : rteventslib/Sources/RTE PWM  ShiftedTransition=Enabled  MaxEvents=4  SampleTime=Ts
  RTE_PWM : Outport
  wires:
  RTE PWM Bot 3/1 -> Bus Creator/6
  RTE PWM Top 3/1 -> Bus Creator/5
  RTE PWM Bot 2/1 -> Bus Creator/4
  RTE PWM Top 2/1 -> Bus Creator/3
  RTE PWM Bot 1/1 -> Bus Creator/2
  RTE PWM Top 1/1 -> Bus Creator/1
  Demux2/6 -> RTE PWM Bot 3/2
  Demux2/5 -> RTE PWM Top 3/2
  Demux2/4 -> RTE PWM Bot 2/2
  Demux2/3 -> RTE PWM Top 2/2
  Demux2/2 -> RTE PWM Bot 1/2
  Demux/6 -> RTE PWM Bot 3/1
  Demux/5 -> RTE PWM Top 3/1
  Demux/3 -> RTE PWM Top 2/1
  Demux/4 -> RTE PWM Bot 2/1
  Demux/2 -> RTE PWM Bot 1/1
  Demux2/1 -> RTE PWM Top 1/2
  Demux/1 -> RTE PWM Top 1/1
  Bus Selector3/2 -> Demux2/1  "<Duty>"
  Bus Selector3/1 -> Demux/1  "<Freq>"
  Bus Creator/1 -> RTE_PWM/1
  PWM_in/1 -> Bus Selector3/1

== system BANSHEE/SS_PV_BESS/EPC/Controller Mapping/RTE Selector ==
  note: MSB
  note: LSB
  In0 : Inport
  In1 : Inport  Port=2
  In2 : Inport  Port=3
  In3 : Inport  Port=4
  In4 : Inport  Port=5
  En : Inport  Port=6
  Bus Selector : BusSelector  OutputSignals=signal1,signal2,signal3,signal4
  RTE Switch{,1..3} (4 alike) : rteventslib/Signal Routing/RTE Switch  switchType=u2 = Double; u1 u3 = RTE Boolean  criteria=u2 >= Threshold  threshold=0.5  interpolate=on  nbMaxEvents=4
  Out : Outport
  wires:
  RTE Switch/1 -> RTE Switch1/1
  RTE Switch1/1 -> RTE Switch2/1
  RTE Switch2/1 -> RTE Switch3/1
  In4/1 -> RTE Switch/1
  In3/1 -> RTE Switch/3
  In2/1 -> RTE Switch1/3
  In1/1 -> RTE Switch2/3
  RTE Switch3/1 -> Out/1
  In0/1 -> RTE Switch3/3
  En/1 -> Bus Selector/1
  Bus Selector/4 -> RTE Switch3/2  "<signal4>"
  Bus Selector/3 -> RTE Switch2/2  "<signal3>"
  Bus Selector/2 -> RTE Switch1/2  "<signal2>"
  Bus Selector/1 -> RTE Switch/2  "<signal1>"

== system BANSHEE/SS_PV_BESS/EPC/Controller Mapping/Signal Mapping ==
  In1 : Inport
  Bus Creator : BusCreator  Inputs=6
  Demux : Demux  Outputs=8
  Out1 : Outport
  wires:
  Demux/1 -> Bus Creator/2  "Phase 1 Bot Switch"
  Demux/2 -> Bus Creator/1  "Phase 1 Top Switch"
  Demux/3 -> Bus Creator/4  "Phase 2 Bot Switch"
  Demux/4 -> Bus Creator/3  "Phase 2 Top Switch"
  Demux/5 -> Bus Creator/6  "Phase 3 Bot Switch"
  Demux/6 -> Bus Creator/5  "Phase 3 Top Switch"
  Bus Creator/1 -> Out1/1  "PWM_RTE"
  In1/1 -> Demux/1

== system BANSHEE/SS_PV_BESS/EPC/Inverter_Batt_RTE/TSB_hiZ snubber_free (contains 6 real diode) ==
  note: Rule of the thumb for Rsnubber=Lload/Ts
      | put maximum R for stability,
      | Then add 1-10 uf typ for Csnubber to make sure current goes to zero after a while
  g : Inport
  Demux5 : Demux  Outputs=[2 2 2]
  MMC_1P1 : Subsystem  mask(MMC cell){Ron=1e-3, Vf=0, Gp=1000/100, Gi=100*0.1e-6, Ts=Ts, dc_short_resistance=10, alt_Idc=off, alt_Idc_comp=.5}
      mask prompts: Ron "Switch conduction resistance [Ohms]"; Vf "Switch conduction voltage offset [V]"; Gp "Snubber resistance (in high impedance mode only) [Ohms]"; Gi "Snubber capacitor (in high impedance mode only) [Farads]"; Ts "Sample time [s]"; dc_short_resistance "Anti-voltage reversal equivalent diode resistance  [Ohms]"; alt_Idc "Alternate Idc calculation method based on power balance"; alt_Idc_comp "Alternate Idc compensation factor (default=0) (0...1)"
      mask help:
      | The MMC cell block implement a unipolar bridge with a capacitor.
      | Series RC snubber circuits are connected in parallel with each switch device.
      |
      | Press Help for suggested snubber values when the model is discretized.
      mask Help: eval('fts2help(''ARTEMiSMMC1PCell'');');
      mask Callback alt_Idc:
      | block=gcb;
      | x=get_param(block,'alt_Idc');
      | y=get_param(block,'MaskVisibilities');
      | if isequal (x,'on')
      |     y{8}='on';
      | else
      |     y{8}='off';
      | end
      | set_param(block,'MaskVisibilities',y);
  MMC_1P2 : Subsystem  mask(MMC cell){Ron=1e-3, Vf=0, Gp=1000/100, Gi=100*0.1e-6, Ts=Ts, dc_short_resistance=10, alt_Idc=off, alt_Idc_comp=.5}
      mask prompts: Ron "Switch conduction resistance [Ohms]"; Vf "Switch conduction voltage offset [V]"; Gp "Snubber resistance (in high impedance mode only) [Ohms]"; Gi "Snubber capacitor (in high impedance mode only) [Farads]"; Ts "Sample time [s]"; dc_short_resistance "Anti-voltage reversal equivalent diode resistance  [Ohms]"; alt_Idc "Alternate Idc calculation method based on power balance"; alt_Idc_comp "Alternate Idc compensation factor (default=0) (0...1)"
      mask help:
      | The MMC cell block implement a unipolar bridge with a capacitor.
      | Series RC snubber circuits are connected in parallel with each switch device.
      |
      | Press Help for suggested snubber values when the model is discretized.
      mask Help: eval('fts2help(''ARTEMiSMMC1PCell'');');
      mask Callback alt_Idc:
      | block=gcb;
      | x=get_param(block,'alt_Idc');
      | y=get_param(block,'MaskVisibilities');
      | if isequal (x,'on')
      |     y{8}='on';
      | else
      |     y{8}='off';
      | end
      | set_param(block,'MaskVisibilities',y);
  MMC_1P3 : Subsystem  mask(MMC cell){Ron=1e-3, Vf=0, Gp=1000/100, Gi=100*0.1e-6, Ts=Ts, dc_short_resistance=10, alt_Idc=off, alt_Idc_comp=.5}
      mask prompts: Ron "Switch conduction resistance [Ohms]"; Vf "Switch conduction voltage offset [V]"; Gp "Snubber resistance (in high impedance mode only) [Ohms]"; Gi "Snubber capacitor (in high impedance mode only) [Farads]"; Ts "Sample time [s]"; dc_short_resistance "Anti-voltage reversal equivalent diode resistance  [Ohms]"; alt_Idc "Alternate Idc calculation method based on power balance"; alt_Idc_comp "Alternate Idc compensation factor (default=0) (0...1)"
      mask help:
      | The MMC cell block implement a unipolar bridge with a capacitor.
      | Series RC snubber circuits are connected in parallel with each switch device.
      |
      | Press Help for suggested snubber values when the model is discretized.
      mask Help: eval('fts2help(''ARTEMiSMMC1PCell'');');
      mask Callback alt_Idc:
      | block=gcb;
      | x=get_param(block,'alt_Idc');
      | y=get_param(block,'MaskVisibilities');
      | if isequal (x,'on')
      |     y{8}='on';
      | else
      |     y{8}='off';
      | end
      | set_param(block,'MaskVisibilities',y);
  + : PMIOPort  Port=1  Side=Right
  A : PMIOPort  Port=2  Side=Left
  - : PMIOPort  Port=3  Side=Right
  B : PMIOPort  Port=4  Side=Left
  C : PMIOPort  Port=5  Side=Left
  wires:
  Demux5/1 -> MMC_1P1/1(g)
  Demux5/2 -> MMC_1P2/1(g)
  Demux5/3 -> MMC_1P3/1(g)
  g/1 -> Demux5/1
  connections:
  A/RConn1 -- MMC_1P1/LConn1
  B/RConn1 -- MMC_1P2/LConn1
  C/RConn1 -- MMC_1P3/LConn1
  MMC_1P3/RConn1 -- +/RConn1 -- MMC_1P1/RConn1 -- MMC_1P2/RConn1
  MMC_1P3/RConn2 -- -/RConn1 -- MMC_1P1/RConn2 -- MMC_1P2/RConn2

== system BANSHEE/SS_PV_BESS/EPC/Inverter_Batt_RTE1/TSB_hiZ snubber_free (contains 6 real diode) ==
  note: Rule of the thumb for Rsnubber=Lload/Ts
      | put maximum R for stability,
      | Then add 1-10 uf typ for Csnubber to make sure current goes to zero after a while
  g : Inport
  Demux5 : Demux  Outputs=[2 2 2]
  MMC_1P1 : Subsystem  mask(MMC cell){Ron=1e-3, Vf=0, Gp=1000/100, Gi=100*0.1e-6, Ts=Ts, dc_short_resistance=10, alt_Idc=off, alt_Idc_comp=.5}
      mask prompts: Ron "Switch conduction resistance [Ohms]"; Vf "Switch conduction voltage offset [V]"; Gp "Snubber resistance (in high impedance mode only) [Ohms]"; Gi "Snubber capacitor (in high impedance mode only) [Farads]"; Ts "Sample time [s]"; dc_short_resistance "Anti-voltage reversal equivalent diode resistance  [Ohms]"; alt_Idc "Alternate Idc calculation method based on power balance"; alt_Idc_comp "Alternate Idc compensation factor (default=0) (0...1)"
      mask help:
      | The MMC cell block implement a unipolar bridge with a capacitor.
      | Series RC snubber circuits are connected in parallel with each switch device.
      |
      | Press Help for suggested snubber values when the model is discretized.
      mask Help: eval('fts2help(''ARTEMiSMMC1PCell'');');
      mask Callback alt_Idc:
      | block=gcb;
      | x=get_param(block,'alt_Idc');
      | y=get_param(block,'MaskVisibilities');
      | if isequal (x,'on')
      |     y{8}='on';
      | else
      |     y{8}='off';
      | end
      | set_param(block,'MaskVisibilities',y);
  MMC_1P2 : Subsystem  mask(MMC cell){Ron=1e-3, Vf=0, Gp=1000/100, Gi=100*0.1e-6, Ts=Ts, dc_short_resistance=10, alt_Idc=off, alt_Idc_comp=.5}
      mask prompts: Ron "Switch conduction resistance [Ohms]"; Vf "Switch conduction voltage offset [V]"; Gp "Snubber resistance (in high impedance mode only) [Ohms]"; Gi "Snubber capacitor (in high impedance mode only) [Farads]"; Ts "Sample time [s]"; dc_short_resistance "Anti-voltage reversal equivalent diode resistance  [Ohms]"; alt_Idc "Alternate Idc calculation method based on power balance"; alt_Idc_comp "Alternate Idc compensation factor (default=0) (0...1)"
      mask help:
      | The MMC cell block implement a unipolar bridge with a capacitor.
      | Series RC snubber circuits are connected in parallel with each switch device.
      |
      | Press Help for suggested snubber values when the model is discretized.
      mask Help: eval('fts2help(''ARTEMiSMMC1PCell'');');
      mask Callback alt_Idc:
      | block=gcb;
      | x=get_param(block,'alt_Idc');
      | y=get_param(block,'MaskVisibilities');
      | if isequal (x,'on')
      |     y{8}='on';
      | else
      |     y{8}='off';
      | end
      | set_param(block,'MaskVisibilities',y);
  MMC_1P3 : Subsystem  mask(MMC cell){Ron=1e-3, Vf=0, Gp=1000/100, Gi=100*0.1e-6, Ts=Ts, dc_short_resistance=10, alt_Idc=off, alt_Idc_comp=.5}
      mask prompts: Ron "Switch conduction resistance [Ohms]"; Vf "Switch conduction voltage offset [V]"; Gp "Snubber resistance (in high impedance mode only) [Ohms]"; Gi "Snubber capacitor (in high impedance mode only) [Farads]"; Ts "Sample time [s]"; dc_short_resistance "Anti-voltage reversal equivalent diode resistance  [Ohms]"; alt_Idc "Alternate Idc calculation method based on power balance"; alt_Idc_comp "Alternate Idc compensation factor (default=0) (0...1)"
      mask help:
      | The MMC cell block implement a unipolar bridge with a capacitor.
      | Series RC snubber circuits are connected in parallel with each switch device.
      |
      | Press Help for suggested snubber values when the model is discretized.
      mask Help: eval('fts2help(''ARTEMiSMMC1PCell'');');
      mask Callback alt_Idc:
      | block=gcb;
      | x=get_param(block,'alt_Idc');
      | y=get_param(block,'MaskVisibilities');
      | if isequal (x,'on')
      |     y{8}='on';
      | else
      |     y{8}='off';
      | end
      | set_param(block,'MaskVisibilities',y);
  + : PMIOPort  Port=1  Side=Right
  A : PMIOPort  Port=2  Side=Left
  - : PMIOPort  Port=3  Side=Right
  B : PMIOPort  Port=4  Side=Left
  C : PMIOPort  Port=5  Side=Left
  wires:
  Demux5/1 -> MMC_1P1/1(g)
  Demux5/2 -> MMC_1P2/1(g)
  Demux5/3 -> MMC_1P3/1(g)
  g/1 -> Demux5/1
  connections:
  A/RConn1 -- MMC_1P1/LConn1
  B/RConn1 -- MMC_1P2/LConn1
  C/RConn1 -- MMC_1P3/LConn1
  MMC_1P3/RConn1 -- +/RConn1 -- MMC_1P1/RConn1 -- MMC_1P2/RConn1
  MMC_1P3/RConn2 -- -/RConn1 -- MMC_1P1/RConn2 -- MMC_1P2/RConn2

== system BANSHEE/SC_ctrl/EPC Inverter/16TSDIn/16 TSDOut GR3/Dout state ctrl/Dout_CH16_CH23 ==
  Bus Creator1 : BusCreator  Inputs=8
  Dout_CH{16..23} (8 alike) : Constant  Value=[1 0 1 0]
  Manual Switch{17..24} (8 alike) : ManualSwitch
  Zero_Dout_CH{16..23} (8 alike) : Constant  Value=[0 0 0 0]
  Dout_CH8_CH15 : Outport
  wires:
  Bus Creator1/1 -> Dout_CH8_CH15/1
  Dout_CH16/1 -> Manual Switch17/1
  Zero_Dout_CH16/1 -> Manual Switch17/2
  Dout_CH17/1 -> Manual Switch18/1
  Zero_Dout_CH17/1 -> Manual Switch18/2
  Dout_CH18/1 -> Manual Switch19/1
  Zero_Dout_CH18/1 -> Manual Switch19/2
  Dout_CH19/1 -> Manual Switch20/1
  Zero_Dout_CH19/1 -> Manual Switch20/2
  Dout_CH20/1 -> Manual Switch21/1
  Zero_Dout_CH20/1 -> Manual Switch21/2
  Dout_CH21/1 -> Manual Switch22/1
  Zero_Dout_CH21/1 -> Manual Switch22/2
  Dout_CH22/1 -> Manual Switch23/1
  Zero_Dout_CH22/1 -> Manual Switch23/2
  Dout_CH23/1 -> Manual Switch24/1
  Zero_Dout_CH23/1 -> Manual Switch24/2
  Manual Switch17/1 -> Bus Creator1/1  "states 17"
  Manual Switch18/1 -> Bus Creator1/2  "states 18"
  Manual Switch19/1 -> Bus Creator1/3  "states 19"
  Manual Switch20/1 -> Bus Creator1/4  "states 20"
  Manual Switch21/1 -> Bus Creator1/5  "states 21"
  Manual Switch22/1 -> Bus Creator1/6  "states 22"
  Manual Switch23/1 -> Bus Creator1/7  "states 23"
  Manual Switch24/1 -> Bus Creator1/8  "states 24"

== system BANSHEE/SC_ctrl/EPC Inverter/16TSDIn/16 TSDOut GR3/Dout state ctrl/Dout_CH24_CH31 ==
  Bus Creator : BusCreator  Inputs=8
  Dout_CH{24..31} (8 alike) : Constant  Value=[1 0 1 0]
  Manual Switch{25..32} (8 alike) : ManualSwitch
  Zero_Dout_CH{24..31} (8 alike) : Constant  Value=[0 0 0 0]
  Dout_CH8_CH15 : Outport
  wires:
  Manual Switch32/1 -> Bus Creator/8  "states 32"
  Manual Switch31/1 -> Bus Creator/7  "states 31"
  Manual Switch30/1 -> Bus Creator/6  "states 30"
  Manual Switch29/1 -> Bus Creator/5  "states 29"
  Manual Switch28/1 -> Bus Creator/4  "states 28"
  Manual Switch27/1 -> Bus Creator/3  "states 27"
  Manual Switch26/1 -> Bus Creator/2  "states 26"
  Manual Switch25/1 -> Bus Creator/1  "states 25"
  Zero_Dout_CH31/1 -> Manual Switch32/2
  Dout_CH31/1 -> Manual Switch32/1
  Zero_Dout_CH30/1 -> Manual Switch31/2
  Dout_CH30/1 -> Manual Switch31/1
  Zero_Dout_CH29/1 -> Manual Switch30/2
  Dout_CH29/1 -> Manual Switch30/1
  Zero_Dout_CH28/1 -> Manual Switch29/2
  Dout_CH28/1 -> Manual Switch29/1
  Zero_Dout_CH27/1 -> Manual Switch28/2
  Dout_CH27/1 -> Manual Switch28/1
  Zero_Dout_CH26/1 -> Manual Switch27/2
  Dout_CH26/1 -> Manual Switch27/1
  Zero_Dout_CH25/1 -> Manual Switch26/2
  Dout_CH25/1 -> Manual Switch26/1
  Zero_Dout_CH24/1 -> Manual Switch25/2
  Dout_CH24/1 -> Manual Switch25/1
  Bus Creator/1 -> Dout_CH8_CH15/1

== system BANSHEE/SM_UtilityService/Banshee_HWCtrl_IOs/Woodward Outputs - Diesel - Gen2/DIO - Gr3/Conditioning1 ==
  In1 : Inport
  Bus Creator : BusCreator  Inputs=8
  Demux : Demux  Outputs=8
  Out1 : Outport
  wires:
  In1/1 -> Demux/1
  Bus Creator/1 -> Out1/1  "DI_CH08-15"
  Demux/8 -> Bus Creator/8  "Gen2_Alarm_CF"
  Demux/7 -> Bus Creator/7  "Gen2_Alarm_AB"
  Demux/6 -> Bus Creator/6  "Gen2_Open_MCB"
  Demux/5 -> Bus Creator/5  "Gen2_Close_MCB"
  Demux/4 -> Bus Creator/4  "Gen2_Open_GCB"
  Demux/3 -> Bus Creator/3  "Gen2_Close_GCB"
  Demux/2 -> Bus Creator/2  "Gen2_Fuel"
  Demux/1 -> Bus Creator/1  "Gen2_Starter"

== system BANSHEE/SM_UtilityService/Banshee_HWCtrl_IOs/Woodward Outputs - Diesel - Gen2/Woodward Primary Inputs - Gen2/Lowpass Filter2 ==
  In : Inport
  Generated Filter Block : DiscreteFir  Tag=BlockMethodSubSystem  Coefficients=[0.0069552863617617106 0.014587901014631248 -0.0057896483056441538 -0.056861876528372622 -0.059476680260783142 0.076118200884714562 0.29579154768342669 0.40638624201187618 0.29579154768342669 0.076118200884714562 -0.059476680260783142 -0.056861876528372622 -0.0057896483056441538 0.014587901014631248 0.0069552863617617106]  InputProcessing=Columns as channels (frame based)
  Out : Outport
  wires:
  In/1 -> Generated Filter Block/1
  Generated Filter Block/1 -> Out/1

== system BANSHEE/SM_UtilityService/Banshee_HWCtrl_IOs/Woodward Outputs - Diesel - Gen2/Woodward Primary Inputs - Gen2/Lowpass Filter3 ==
  In : Inport
  Generated Filter Block : DiscreteFir  Tag=BlockMethodSubSystem  Coefficients=[0.0069552863617617106 0.014587901014631248 -0.0057896483056441538 -0.056861876528372622 -0.059476680260783142 0.076118200884714562 0.29579154768342669 0.40638624201187618 0.29579154768342669 0.076118200884714562 -0.059476680260783142 -0.056861876528372622 -0.0057896483056441538 0.014587901014631248 0.0069552863617617106]  InputProcessing=Columns as channels (frame based)
  Out : Outport
  wires:
  In/1 -> Generated Filter Block/1
  Generated Filter Block/1 -> Out/1

== system BANSHEE/SM_UtilityService/Banshee_HWCtrl_IOs/Woodward Outputs - NGCHP - Gen1/DIO - Gr3/Conditioning ==
  In1 : Inport
  Bus Creator : BusCreator  Inputs=8
  Demux : Demux  Outputs=8
  Out1 : Outport
  wires:
  Demux/1 -> Bus Creator/1  "Gen1_Starter"
  Demux/2 -> Bus Creator/2  "Gen1_Fuel"
  Demux/3 -> Bus Creator/3  "Gen1_Close_GCB"
  Demux/4 -> Bus Creator/4  "Gen1_Open_GCB"
  Demux/5 -> Bus Creator/5  "Gen1_Close_MCB"
  Demux/6 -> Bus Creator/6  "Gen1_Open_MCB"
  Demux/7 -> Bus Creator/7  "Gen1_Alarm_AB"
  Demux/8 -> Bus Creator/8  "Gen1_Alarm_CF"
  Bus Creator/1 -> Out1/1  "DI_CH00-07"
  In1/1 -> Demux/1

== system BANSHEE/SM_UtilityService/Banshee_HWCtrl_IOs/Woodward Outputs - NGCHP - Gen1/Woodward Primary Inputs - Gen1/Lowpass Filter ==
  In : Inport
  Generated Filter Block : DiscreteFir  Tag=BlockMethodSubSystem  Coefficients=[0.0069552863617617106 0.014587901014631248 -0.0057896483056441538 -0.056861876528372622 -0.059476680260783142 0.076118200884714562 0.29579154768342669 0.40638624201187618 0.29579154768342669 0.076118200884714562 -0.059476680260783142 -0.056861876528372622 -0.0057896483056441538 0.014587901014631248 0.0069552863617617106]  InputProcessing=Columns as channels (frame based)
  Out : Outport
  wires:
  In/1 -> Generated Filter Block/1
  Generated Filter Block/1 -> Out/1

== system BANSHEE/SM_UtilityService/Banshee_HWCtrl_IOs/Woodward Outputs - NGCHP - Gen1/Woodward Primary Inputs - Gen1/Lowpass Filter1 ==
  In : Inport
  Generated Filter Block : DiscreteFir  Tag=BlockMethodSubSystem  Coefficients=[0.0069552863617617106 0.014587901014631248 -0.0057896483056441538 -0.056861876528372622 -0.059476680260783142 0.076118200884714562 0.29579154768342669 0.40638624201187618 0.29579154768342669 0.076118200884714562 -0.059476680260783142 -0.056861876528372622 -0.0057896483056441538 0.014587901014631248 0.0069552863617617106]  InputProcessing=Columns as channels (frame based)
  Out : Outport
  wires:
  In/1 -> Generated Filter Block/1
  Generated Filter Block/1 -> Out/1

== system BANSHEE/SS_PV_BESS/EPC/Controller Mapping/6-pulse RTE PWM generator (with deadtime)/Discrete Triangular-Waveform Generator ==
  Constant : Constant  Value=Vpeak
  Constant1 : Constant  Value=NumberSteps
  Constant2 : Constant  Value=Freq_used
  Fcn2 : Fcn  Expr=u[2]/u[1]
  Fcn3 : Fcn  Expr=4 *u[1] -1
  Fcn4 : Fcn  Expr=-4 *u[1] +3
  Fd1 : Constant  Value=-1
  Fd2 : Constant
  Fd4 : Constant
  Gain1 : Gain  Gain=1/2  SaturateOnIntegerOverflow=on  OutDataTypeStr=Inherit: Same as input  ParamDataTypeStr=Inherit: Same as input
  Mux5 : Mux  Inputs=2
  Product : Product  SaturateOnIntegerOverflow=on  InputSameDT=on  OutDataTypeStr=Inherit: Same as first input
  Relational Operator1 : RelationalOperator  Operator=>  InputSameDT=on
  Relational Operator2 : RelationalOperator  Operator===  InputSameDT=on
  Sum : Sum  SaturateOnIntegerOverflow=on  InputSameDT=on  OutDataTypeStr=Inherit: Same as first input
  Sum2 : Sum  Inputs=+-  SaturateOnIntegerOverflow=on  InputSameDT=on  OutDataTypeStr=Inherit: Same as first input
  Switch : Switch  Threshold=0.5  SaturateOnIntegerOverflow=on  InputSameDT=on
  Switch1 : Switch  Threshold=0.5  SaturateOnIntegerOverflow=on  InputSameDT=on
  Unit Delay : UnitDelay  SampleTime=Ts
  Unit Delay1 : UnitDelay  SampleTime=Ts
  Triangle : Outport  InitialOutput=0
  Freq_used : Outport  Port=2  InitialOutput=0
  wires:
  Constant2/1 -> Freq_used/1
  Relational Operator1/1 -> Switch1/2
  Gain1/1 -> Relational Operator1/2
  Fcn3/1 -> Switch1/3
  Fcn4/1 -> Switch1/1
  Mux5/1 -> Fcn2/1
  Fcn2/1 -> Fcn3/1, Fcn4/1
  Sum/1 -> Mux5/2, Relational Operator1/1, Relational Operator2/2, Unit Delay/1
  Constant1/1 -> Gain1/1, Mux5/1, Sum2/1
  Sum2/1 -> Relational Operator2/1
  Relational Operator2/1 -> Unit Delay1/1
  Unit Delay1/1 -> Switch/2
  Unit Delay/1 -> Switch/3
  Fd1/1 -> Switch/1
  Fd2/1 -> Sum/2
  Switch/1 -> Sum/1
  Fd4/1 -> Sum2/2
  Constant/1 -> Product/1
  Switch1/1 -> Product/2
  Product/1 -> Triangle/1

== system BANSHEE/SS_PV_BESS/EPC/Controller Mapping/EPC Inverter Controller Outputs/DIO - Gr4 ==
  Dout : Inport
  Bus Creator : BusCreator  Inputs=2
  Bus Selector : BusSelector  OutputSignals=DI_CH00-07  OutputAsBus=on
  Bus Selector1 : BusSelector  OutputSignals=DI_CH08-15  OutputAsBus=on
  Conditioning : Subsystem
  Conditioning1 : Subsystem
  OP5142EX2 DigitalIn : rtio_opalrt_op5142ex1/OP5142EX1 DigitalIn  CtrlName='OP5142EX2 Ctrl'  portNb=3  FcnNos=Slot 4 Module A Subsection 1  size=1  maxcount=8  count=8  sampleTime=0  numchan=8
      settings: AttributesFormatString=%<CtrlName>
  OP5142EX2 DigitalIn1 : rtio_opalrt_op5142ex1/OP5142EX1 DigitalIn  CtrlName='OP5142EX2 Ctrl'  portNb=4  FcnNos=Slot 4 Module A Subsection 2  size=1  maxcount=8  count=8  sampleTime=0  numchan=8
      settings: AttributesFormatString=%<CtrlName>
  OP5142EX2 DigitalOut : rtio_opalrt_op5142ex1/OP5142EX1 DigitalOut  CtrlName='OP5142EX2 Ctrl'  portNb=9  FcnNos=Slot 4 Module B Subsection 1  size=1  maxcount=8  count=8  numchan=8
      settings: AttributesFormatString=%<CtrlName>
  OP5142EX2 DigitalOut1 : rtio_opalrt_op5142ex1/OP5142EX1 DigitalOut  CtrlName='OP5142EX2 Ctrl'  portNb=10  FcnNos=Slot 4 Module B Subsection 2  size=1  maxcount=8  count=8  numchan=8
      settings: AttributesFormatString=%<CtrlName>
  Terminator{1,3,5..6} (4 alike) : Terminator
  DIn : Outport
  wires:
  OP5142EX2 DigitalOut/1 -> Terminator3/1
  OP5142EX2 DigitalOut1/1 -> Terminator1/1
  Dout/1 -> Bus Selector/1, Bus Selector1/1
  Bus Selector/1 -> OP5142EX2 DigitalOut/1
  Bus Selector1/1 -> OP5142EX2 DigitalOut1/1
  OP5142EX2 DigitalIn/2 -> Terminator5/1
  OP5142EX2 DigitalIn1/2 -> Terminator6/1
  OP5142EX2 DigitalIn/1 -> Conditioning/1(In1)  "DI_CH00-07"
  OP5142EX2 DigitalIn1/1 -> Conditioning1/1(In1)  "DI_CH08-15"
  Bus Creator/1 -> DIn/1
  Conditioning/1(Out1) -> Bus Creator/1
  Conditioning1/1(Out1) -> Bus Creator/2

== system BANSHEE/SS_PV_BESS/EPC/Controller Mapping/EPC Inverter Controller Outputs/DOUT type config ==
  note: The Constants are used to select Digital Output type:
      | - 0: Time-Stamped Digital Output
      | - 1: Pulse-Width Modulated DIgital Output
  OP5142EX2 DataIn Send : rtio_opalrt_op5142ex1/OP5142EX1 DataIn Send  CtrlName='OP5142EX2 Ctrl'  FcnNosp1=15  FcnNos=-1  FcnNosm1=(15)-1  width=1  portType=double  numwidth=1
      settings: AttributesFormatString=%<CtrlName>
  OP5142EX2 DataIn Send1 : rtio_opalrt_op5142ex1/OP5142EX1 DataIn Send  CtrlName='OP5142EX2 Ctrl'  FcnNosp1=16  FcnNos=-1  FcnNosm1=(16)-1  width=1  portType=double  numwidth=1
      settings: AttributesFormatString=%<CtrlName>
  Subsection 3 DOUT type : Constant  Value=0
  Subsection 4 DOUT type : Constant  Value=0
  Terminator1 : Terminator
  Terminator2 : Terminator
  wires:
  Subsection 3 DOUT type/1 -> OP5142EX2 DataIn Send/1
  Subsection 4 DOUT type/1 -> OP5142EX2 DataIn Send1/1
  OP5142EX2 DataIn Send1/1 -> Terminator1/1
  OP5142EX2 DataIn Send/1 -> Terminator2/1

== system BANSHEE/SS_PV_BESS/EPC/Controller Mapping/EPC Inverter Controller Outputs/GR1 B AIN (CH00-15) ==
  Mux6 : Mux  Inputs=2
  OP5142EX2 AnalogIn : rtio_opalrt_op5142ex1/OP5142EX1 AnalogIn  CtrlName='OP5142EX2 Ctrl'  portNb=1  FcnNos=Slot 1 Module B Subsection 1  size=16  maxcount=8  count=8  numchan=8  sampleTime=0
      settings: AttributesFormatString=%<CtrlName>
  OP5142EX2 AnalogIn1 : rtio_opalrt_op5142ex1/OP5142EX1 AnalogIn  CtrlName='OP5142EX2 Ctrl'  portNb=2  FcnNos=Slot 1 Module B Subsection 2  size=16  maxcount=8  count=8  numchan=8  sampleTime=0
      settings: AttributesFormatString=%<CtrlName>
  Terminator2 : Terminator
  Terminator3 : Terminator
  Ain : Outport
  wires:
  Mux6/1 -> Ain/1
  OP5142EX2 AnalogIn1/2 -> Terminator3/1
  OP5142EX2 AnalogIn/2 -> Terminator2/1
  OP5142EX2 AnalogIn1/1 -> Mux6/2
  OP5142EX2 AnalogIn/1 -> Mux6/1
